simulink model "Qmod3"
settings: Solver=ode45  StartTime=0.0  StopTime=10.0  RelTol=1e-3
values from neighbouring files (symbols this model uses):
  g = 9.81    [Qconst.m]
  Ixx = 1    [Qconst.m]
  Iyy = 1    [Qconst.m]
  Izz = 1    [Qconst.m]
  k = 1    [Qconst.m]
  l = 1    [Qconst.m]
  m = 1    [Qconst.m]
settings Model: Creator=DNI 38876767  LastModifiedBy=gabriel
settings DataIOCC: LimitDataPoints=on  SaveFormat=Array  ReturnWorkspaceOutputs=off
settings OptimizationCC: ExpressionDepthLimit=2147483647  LifeSpan=inf  SimCompilerOptimization=Off
settings DebuggingCC: UnderspecifiedInitializationDetection=Classic  MergeDetectMultiDrivingBlocksExec=none  SolverPrmCheckMsg=warning  MultiTaskDSMMsg=warning  MultiTaskCondExecSysMsg=none  FcnCallInpInsideContextMsg=Enable All  FrameProcessingCompatibilityMsg=warning  StateNameClashWarn=warning  StrictBusMsg=None  SFUnexpectedBacktrackingDiag=warning  SFNoUnconditionalDefaultTransitionDiag=warning
settings HardwareCC: ProdBitPerPointer=32  ProdLargestAtomicFloat=None  ProdIntDivRoundTo=Undefined  ProdEndianess=Unspecified  ProdWordSize=32  ProdHWDeviceType=32-bit Generic
settings ModelReferenceCC: PropagateSignalLabelsOutOfModel=off
settings SFSimCC: SimUseLocalCustomCode=off
settings RTWCC: RTWUseLocalCustomCode=off  IncludeERTFirstTime=on  RTWCompilerOptimization=Off
settings CodeAppCC: CustomSymbolStrType=$N$R$M
settings GRTTargetCC: CodeReplacementLibrary=ANSI_C  GeneratePreprocessorConditionals=Disable all  CPPClassGenCompliant=off

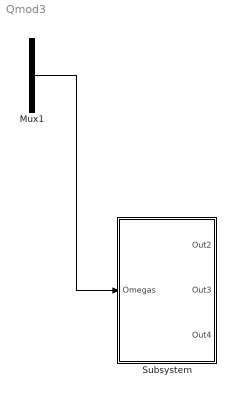
== system Qmod3 ==
  Mux1 : Mux
  Subsystem : Subsystem
  wires:
  Mux1/1 -> Subsystem/1("Omegas ")

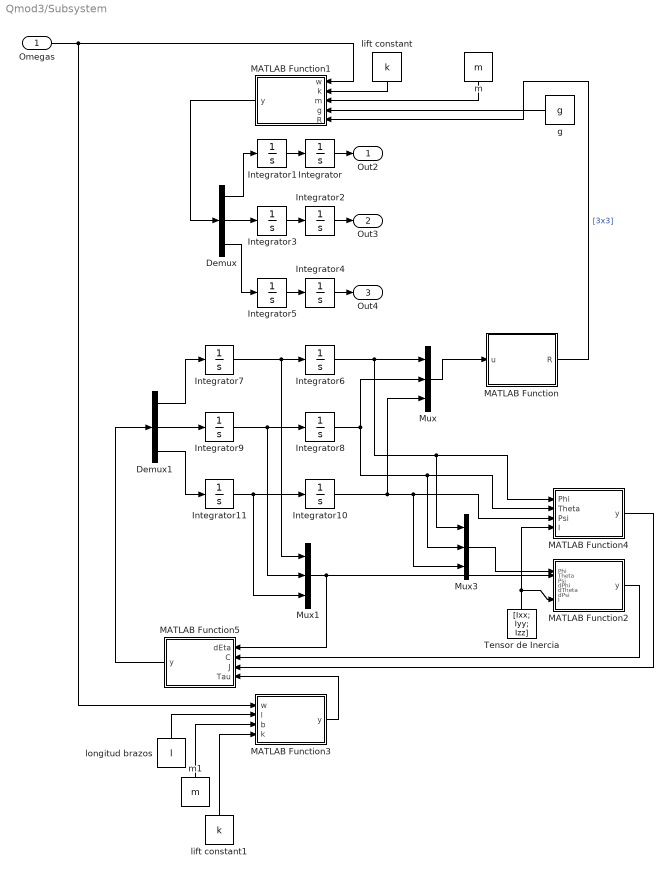
== system Qmod3/Subsystem ==
  "Omegas " : Inport
  Demux : Demux  Outputs=3
  Demux1 : Demux  Outputs=3
  Integrator{,2..11} (11 alike) : Integrator
  Integrator1 : Integrator  InitialCondition=1
  MATLAB Function : MATLAB Function  TreatAsAtomicUnit=on
  MATLAB Function1 : MATLAB Function  TreatAsAtomicUnit=on
  MATLAB Function2 : MATLAB Function  TreatAsAtomicUnit=on
  MATLAB Function3 : MATLAB Function  TreatAsAtomicUnit=on
  MATLAB Function4 : MATLAB Function  TreatAsAtomicUnit=on
  MATLAB Function5 : MATLAB Function  TreatAsAtomicUnit=on
  Mux : Mux  Inputs=3
  Mux1 : Mux  Inputs=3
  Mux3 : Mux  Inputs=3
  Tensor de Inercia : Constant  Value=[Ixx; Iyy; Izz]
  g : Constant  Value=g
  lift constant : Constant  Value=k
  lift constant1 : Constant  Value=k
  longitud brazos : Constant  Value=l
  m : Constant  Value=m
  m1 : Constant  Value=m
  Out2 : Outport
  Out3 : Outport  Port=2
  Out4 : Outport  Port=3
  wires:
  Integrator9/1 -> Integrator8/1, Mux1/2
  MATLAB Function1/1(y) -> Demux/1
  Integrator11/1 -> Integrator10/1, Mux1/3
  Integrator5/1 -> Integrator4/1
  Integrator7/1 -> Integrator6/1, Mux1/1
  Integrator3/1 -> Integrator2/1
  Integrator/1 -> Out2/1
  Demux1/1 -> Integrator7/1
  MATLAB Function/1(R) -> MATLAB Function1/5(R)  "[3x3]"
  Integrator4/1 -> Out4/1
  Demux1/3 -> Integrator11/1
  Integrator2/1 -> Out3/1
  Demux1/2 -> Integrator9/1
  "Omegas "/1 -> MATLAB Function3/1(w), MATLAB Function1/1(w)
  Demux/3 -> Integrator5/1
  Integrator8/1 -> Mux3/2, MATLAB Function4/2(Theta), Mux/2
  Mux/1 -> MATLAB Function/1(u)
  Demux/1 -> Integrator1/1
  Demux/2 -> Integrator3/1
  Integrator1/1 -> Integrator/1
  Integrator10/1 -> Mux3/3, MATLAB Function4/3(Psi), Mux/3
  Integrator6/1 -> Mux3/1, MATLAB Function4/1(Phi), Mux/1
  lift constant/1 -> MATLAB Function1/2(k)
  m/1 -> MATLAB Function1/3(m)
  g/1 -> MATLAB Function1/4(g)
  Mux1/1 -> MATLAB Function5/1(dEta), MATLAB Function2/2(Theta)
  Tensor de Inercia/1 -> MATLAB Function4/4(I), MATLAB Function2/7(I)
  longitud brazos/1 -> MATLAB Function3/2(l)
  m1/1 -> MATLAB Function3/3(b)
  lift constant1/1 -> MATLAB Function3/4(k)
  MATLAB Function2/1(y) -> MATLAB Function5/2(C)
  MATLAB Function4/1(y) -> MATLAB Function5/3(J)
  MATLAB Function3/1(y) -> MATLAB Function5/4(Tau)
  MATLAB Function5/1(y) -> Demux1/1
  Mux3/1 -> MATLAB Function2/1(Phi)

== matlab function Qmod3/Subsystem/MATLAB Function1 ==
  data: w input; k input; m input; g input; y output; R input
function y = fcn(w,k,m,g,R)
%#codegen
%k=1;
%eml.extrinsic('k');
Thrust=[0; 0; k*(w(1)+w(2)+w(3)+w(4))/m];
%y = R*Thrust;
y=R*Thrust-[0; 0; -g];

== matlab function Qmod3/Subsystem/MATLAB Function ==
  data: u input; R output
function R = fcn(u)
%#codegen
%H=sym('H')
Phi=u(1);
Theta=u(2);
Psi=u(3);

R = [[cos(Psi)*cos(Theta) cos(Psi)*sin(Theta)*sin(Phi)-sin(Psi)*cos(Phi) cos(Psi)*sin(Theta)*cos(Phi)+sin(Psi)*sin(Phi)];
     [sin(Psi)*cos(Theta) sin(Psi)*sin(Theta)*sin(Phi)+cos(Psi)*cos(Phi) sin(Psi)*sin(Theta)*cos(Phi)-cos(Psi)*sin(Phi)];
     [-sin(Theta) cos(Theta)*sin(Phi) cos(Theta)*cos(Phi)]];

== matlab function Qmod3/Subsystem/MATLAB Function2 ==
  data: Phi input; y output; Theta input; Psi input; dPhi input; dTheta input; dPsi input; I input
function y = fcn(Phi,Theta,Psi,dPhi,dTheta,dPsi,I)
%#codegen

Ixx=I(1);
Iyy=I(2);
Izz=I(3);

C11=0;
C12=(Iyy-Izz)*(dTheta*cos(Phi)*sin(Phi)+dPsi*(sin(Phi)^2)*cos(Theta))+(Izz-Iyy)*dPsi*(cos(Phi)^2)*cos(Theta)-Ixx*dPsi*cos(Theta);
C13=(Izz-Iyy)*dPsi*cos(Phi)*sin(Phi)*(cos(Theta)^2);

% C21=(Izz-Iyy)*(dTheta*cos(Phi)*sin(Phi)+dPsi*(sin(Phi)^2)*cos(Theta))+(Izz-Iyy)*dPsi*(cos(Phi)^2)*cos(Theta)-Ixx*dPsi*cos(Theta);
C21=(Izz-Iyy)*(dTheta*cos(Phi)*sin(Phi)+dPsi*sin(Phi)*cos(Theta))+(Iyy-Izz)*dPsi*(cos(Phi)^2)*cos(Theta)+Ixx*dPsi*cos(Theta);
C22=(Izz-Iyy)*dPhi*cos(Phi)*sin(Phi);
C23=-Ixx*dPsi*sin(Theta)*cos(Theta)+Iyy*dPhi*(sin(Phi)^2)*sin(Theta)*cos(Theta)+Izz*dPsi*(cos(Phi)^2)*sin(Theta)*cos(Theta);

C31=(Iyy-Izz)*dPsi*(cos(Theta)^2)*sin(Phi)*cos(Phi)-Ixx*dTheta*cos(Theta);
C32=(Izz-Iyy)*(dTheta*cos(Phi)*sin(Phi)*sin(Theta)+dPhi*(sin(Phi)^2)*cos(Theta))+(Iyy-Izz)*dPhi*(cos(Phi)^2)*cos(Theta)+Ixx*dPsi*sin(Theta)*cos(Theta)-Iyy*dPsi*(sin(Phi)^2)*sin(Theta)*cos(Theta)-Izz*dPsi*(cos(Phi)^2)*sin(Theta)*cos(Theta);
C33=(Iyy-Izz)*dPhi*cos(Phi)^sin(Phi)*(cos(Theta)^2)-Iyy*dTheta*(sin(Phi)^2)*cos(Theta)*sin(Theta)-Izz*dTheta*(cos(Phi)^2)*cos(Theta)*sin(Theta)+Ixx*dTheta*cos(Theta)*sin(Theta);

C=[[C11 C12 C13];
   [C21 C22 C23];
   [C31 C32 C33]];
y = 1;

== matlab function Qmod3/Subsystem/MATLAB Function3 ==
  data: w input; l input; y output; b input; k input
function y = fcn(w,l,b,k)
%#codegen

y = [l*k*(w(4)^2-w(2)^2);
     l*k*(w(3)^2 - w(1)^2);
     b*(w(1)^2-w(2)^2+w(3)^2-w(4)^2)];

== matlab function Qmod3/Subsystem/MATLAB Function4 ==
  data: Phi input; Theta input; Psi input; y output; I input
function y = fcn(Phi,Theta,Psi,I)
%#codegen



Ixx=I(1);
Iyy=I(2);
Izz=I(3);

Weta=[[1 0 -sin(Theta)];
      [0 cos(Phi) cos(Theta)*sin(Phi)];
      [0 -sin(Phi) cos(Theta)*cos(Phi)]]
  
WetaT=transpose(Weta);

II=[[Ixx 0 0];[0 Iyy 0];[0 0 Izz]];

y = WetaT*II*Weta;

== matlab function Qmod3/Subsystem/MATLAB Function5 ==
  data: dEta input; y output; C input; J input; Tau input
function y = fcn(dEta,C,J,Tau)
%#codegen

y = u;
